simulink model "time_test2"  (R2018b)
settings: Solver=VariableStepAuto  StartTime=0.0  StopTime=0  FixedStep=.2  RelTol=1e-3
values from neighbouring files (symbols this model uses):
  GPS_time = [129600; 2034]    [time_versus_test_init.m]
  t0 = simParams.time.epoch_utc_s    [time_versus_test_init.m]
undefined symbols (not defined in the file or in its folder): clock_lib, GPS_time_lib, simParams, time_coord_rotation_lib
libraries: coord_rotation_lib x1, time_conversion_lib x1, time_Lib x1
settings Model: Creator=devantormey  LastModifiedBy=devantormey

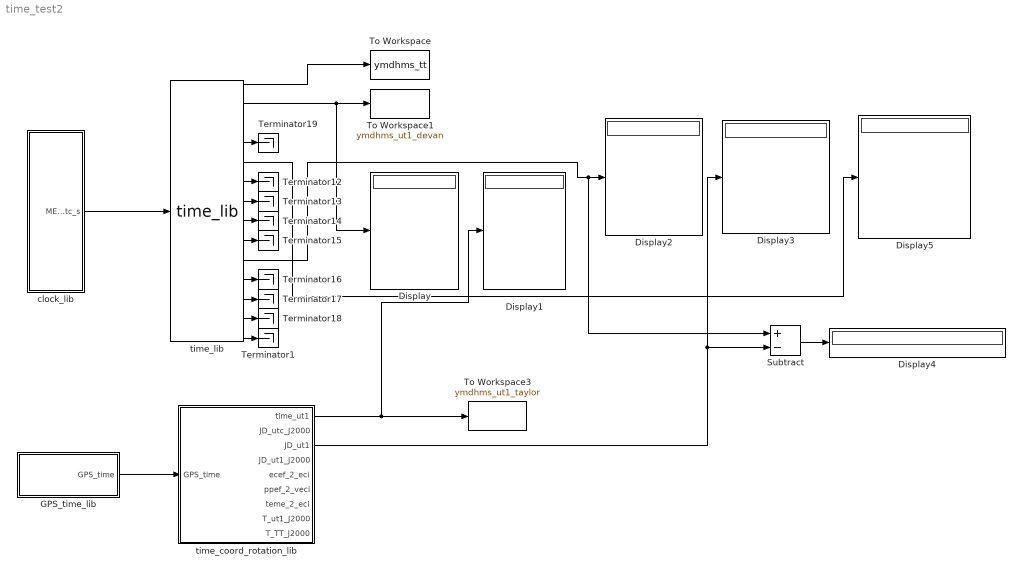
== system time_test2 ==
  Display{,1..5} (6 alike) : Display
  GPS_time_lib : Subsystem  AncestorBlock=GPS_time_lib/GPS_time_lib
  Subtract : Sum  Inputs=+-
  Terminator{1,12..19} (9 alike) : Terminator
  To Workspace : ToWorkspace  VariableName=ymdhms_tt  SaveFormat=Timeseries  SampleTime=-1
  To Workspace1 : ToWorkspace  VariableName=ymdhms_ut1_devan  SaveFormat=Timeseries  SampleTime=-1
  To Workspace3 : ToWorkspace  VariableName=ymdhms_ut1_taylor  SaveFormat=Timeseries  SampleTime=-1
  clock_lib : Subsystem  AncestorBlock=clock_lib/clock_lib
  time_coord_rotation_lib : Subsystem  AncestorBlock=time_coord_rotation_lib/time_coord_rotation_lib
  "time_lib " : time_Lib/time_lib    SystemSampleTime=-1
  wires:
  "time_lib "/8 -> Terminator14/1
  "time_lib "/4 -> Terminator19/1
  "time_lib "/5 -> Display5/1
  "time_lib "/7 -> Terminator13/1
  "time_lib "/11 -> Terminator16/1
  "time_lib "/9 -> Terminator15/1
  "time_lib "/13 -> Terminator18/1
  "time_lib "/6 -> Terminator12/1
  clock_lib/1(MET_utc_s) -> "time_lib "/1
  "time_lib "/2 -> Display/1, To Workspace1/1
  "time_lib "/12 -> Terminator17/1
  "time_lib "/14 -> Terminator1/1
  "time_lib "/1 -> To Workspace/1
  GPS_time_lib/1(GPS_time) -> time_coord_rotation_lib/1(GPS_time)
  time_coord_rotation_lib/1(time_ut1) -> Display1/1, To Workspace3/1
  time_coord_rotation_lib/3(JD_ut1) -> Subtract/2, Display3/1
  "time_lib "/10 -> Subtract/1, Display2/1
  Subtract/1 -> Display4/1

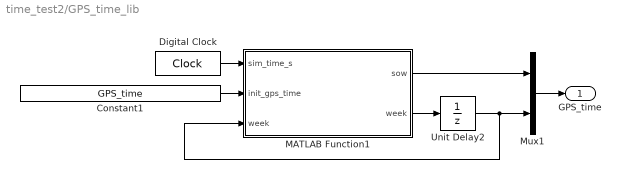
== system time_test2/GPS_time_lib ==
  Constant1 : Constant  Value=GPS_time  VectorParams1D=off  SampleTime=-1
  Digital Clock : DigitalClock  SampleTime=.1
  MATLAB Function1 : MATLAB Function  TreatAsAtomicUnit=on
  Mux1 : Mux  Inputs=2
  Unit Delay2 : UnitDelay  InitialCondition=GPS_time(2)  SampleTime=-1
  GPS_time : Outport
  wires:
  Mux1/1 -> GPS_time/1
  MATLAB Function1/1(sow) -> Mux1/1
  Unit Delay2/1 -> Mux1/2, MATLAB Function1/3("week ")
  MATLAB Function1/2(week) -> Unit Delay2/1
  Constant1/1 -> MATLAB Function1/2(init_gps_time)
  Digital Clock/1 -> MATLAB Function1/1(sim_time_s)

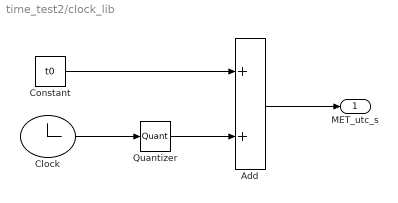
== system time_test2/clock_lib ==
  Add : Sum
  Clock : Clock
  Constant : Constant  Value=t0
  Quantizer : Quantizer  QuantizationInterval=simParams.time.res
  MET_utc_s : Outport
  wires:
  Add/1 -> MET_utc_s/1
  Quantizer/1 -> Add/2
  Constant/1 -> Add/1
  Clock/1 -> Quantizer/1

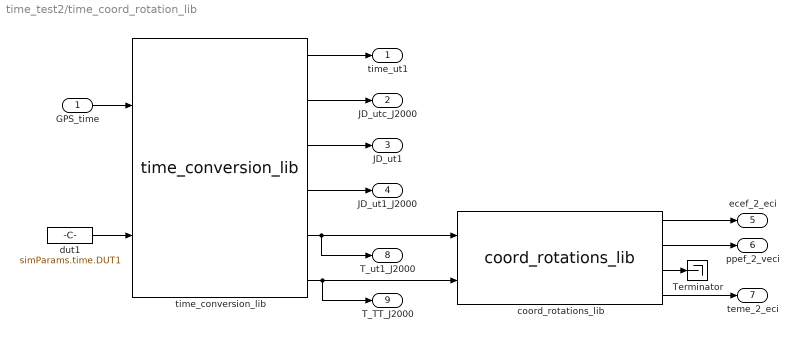
== system time_test2/time_coord_rotation_lib ==
  GPS_time : Inport
  Terminator : Terminator
  coord_rotations_lib : coord_rotation_lib/coord_rotations_lib  SystemSampleTime=-1
  dut1 : Constant  Value=simParams.time.DUT1
  time_conversion_lib : time_conversion_lib/time_conversion_lib  SystemSampleTime=-1
  time_ut1 : Outport
  JD_utc_J2000 : Outport  Port=2
  JD_ut1 : Outport  Port=3
  JD_ut1_J2000 : Outport  Port=4
  ecef_2_eci : Outport  Port=5
  ppef_2_veci : Outport  Port=6
  teme_2_eci : Outport  Port=7
  T_ut1_J2000 : Outport  Port=8
  T_TT_J2000 : Outport  Port=9
  wires:
  dut1/1 -> time_conversion_lib/2
  time_conversion_lib/5 -> T_ut1_J2000/1, coord_rotations_lib/1
  time_conversion_lib/6 -> T_TT_J2000/1, coord_rotations_lib/2
  time_conversion_lib/1 -> time_ut1/1
  time_conversion_lib/3 -> JD_ut1/1
  time_conversion_lib/4 -> JD_ut1_J2000/1
  coord_rotations_lib/1 -> ecef_2_eci/1
  coord_rotations_lib/2 -> ppef_2_veci/1
  coord_rotations_lib/4 -> teme_2_eci/1
  coord_rotations_lib/3 -> Terminator/1
  time_conversion_lib/2 -> JD_utc_J2000/1
  GPS_time/1 -> time_conversion_lib/1

== matlab function time_test2/GPS_time_lib/MATLAB Function1 ==
  data: sim_time_s input; sow output; init_gps_time input; week input; week output
function [sow, week] = gps_clock(sim_time_s, init_gps_time, week)
% ----------------------------------------------------------------------- %
% UW HuskySat-1, ADCS Subsystem
%
% GPS clock for the SIM.
% ----------------------------------------------------------------------- %

% Constants
sec_in_week = 604800;


init_sow    = init_gps_time(1);
sow         = mod(init_sow + sim_time_s, sec_in_week);

% Handle roll overs
if sow == sec_in_week
    week = week + 1;
end

end
